simulink model "KalmanFilter_Lateral"  (R2016b)
settings: Solver=VariableStepAuto  StartTime=0.0  StopTime=100  RelTol=1e-3
undefined symbols (not defined in the file or in its folder): A_lat, B_lat, C_lat, Continuous, D_lat, Time
libraries: ctrlSharedLib x1
settings Model: Creator=yashm  LastModifiedBy=yashm

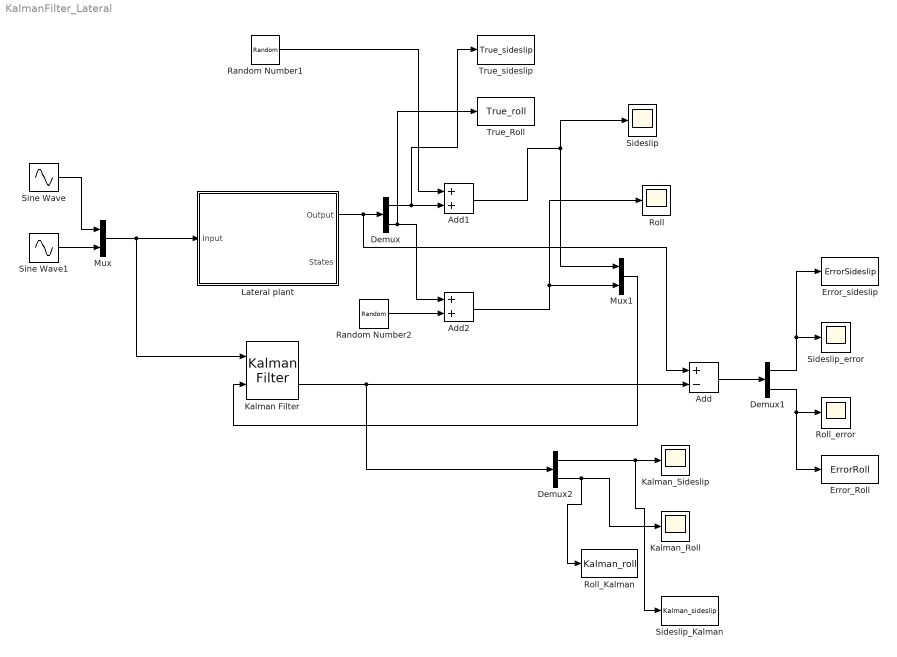
== system KalmanFilter_Lateral ==
  Add : Sum  Inputs=+-
  Add1 : Sum
  Add2 : Sum
  Demux : Demux  Outputs=2
  Demux1 : Demux  Outputs=2
  Demux2 : Demux  Outputs=2
  Error_Roll : ToWorkspace  VariableName=ErrorRoll  SampleTime=0.001
      settings: Save2DSignal=2-D array (concatenate along first dimension)
  Error_sideslip : ToWorkspace  VariableName=ErrorSideslip  SampleTime=0.001
      settings: Save2DSignal=2-D array (concatenate along first dimension)
  Kalman Filter : ctrlSharedLib/Kalman Filter  TimeDomain=Continuous-Time  UseCurrentEstimator=on  ModelSource=Individual A, B, C, D matrices  ModelSourceVariable=ss(0.95,1,1,0,1)  A=A_lat  B=B_lat  C=C_lat  D=D_lat  NumberOfStates=1  NumberOfInputs=1  NumberOfOutputs=1  InitialEstimateSource=Dialog  X0=0  P0=10  UseK=off  UseGH=off  NumberOfProcessNoiseInputs=1  G=1  TimeInvariantG=on  H=0  TimeInvariantH=on  Q=1  TimeInvariantQ=on  R=[1 0;0 1]  TimeInvariantR=on  N=0  TimeInvariantN=on  AddInputPort=on  AddEnablePort=off  ExternalReset=none  OutputEstimatedY=on  OutputP=off  Ts=-1
  Kalman_Roll : Scope
  Kalman_Sideslip : Scope
  "Lateral plant " : Subsystem
  Mux : Mux  Inputs=2
  Mux1 : Mux  Inputs=2
  Random Number1 : RandomNumber  Variance=0.01  SampleTime=0.0001
  Random Number2 : RandomNumber  Variance=3  SampleTime=0.0001
  Roll : Scope
  Roll_Kalman : ToWorkspace  VariableName=Kalman_roll  SampleTime=0.001
      settings: Save2DSignal=2-D array (concatenate along first dimension)
  Roll_error : Scope
  Sideslip : Scope
  Sideslip_Kalman : ToWorkspace  VariableName=Kalman_sideslip  SampleTime=0.001
      settings: Save2DSignal=2-D array (concatenate along first dimension)
  Sideslip_error : Scope
  Sine Wave : Sin  Frequency=15  SampleTime=0
  Sine Wave1 : Sin  Frequency=15  SampleTime=0
  True_Roll : ToWorkspace  VariableName=True_roll  SampleTime=0.001
      settings: Save2DSignal=2-D array (concatenate along first dimension)
  True_sideslip : ToWorkspace  VariableName=True_sideslip  SampleTime=0.001
      settings: Save2DSignal=2-D array (concatenate along first dimension)
  wires:
  "Lateral plant "/1(Output) -> Add/1, Demux/1
  Demux/1 -> True_sideslip/1, Add1/2
  Random Number1/1 -> Add1/1
  Add1/1 -> Mux1/1, Sideslip/1
  Sine Wave1/1 -> Mux/2
  Sine Wave/1 -> Mux/1
  Mux/1 -> Kalman Filter/1, "Lateral plant "/1(Input)
  Kalman Filter/2 -> Demux2/1, Add/2
  Random Number2/1 -> Add2/2
  Demux/2 -> True_Roll/1, Add2/1
  Add2/1 -> Mux1/2, Roll/1
  Mux1/1 -> Kalman Filter/2
  Add/1 -> Demux1/1
  Demux2/1 -> Sideslip_Kalman/1, Kalman_Sideslip/1
  Demux2/2 -> Roll_Kalman/1, Kalman_Roll/1
  Demux1/2 -> Error_Roll/1, Roll_error/1
  Demux1/1 -> Error_sideslip/1, Sideslip_error/1

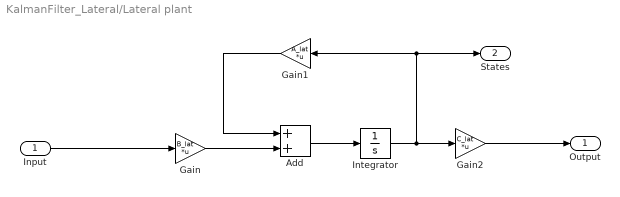
== system KalmanFilter_Lateral/Lateral plant  ==
  Input : Inport
  Add : Sum
  Gain : Gain  Gain=B_lat  Multiplication=Matrix(K*u)
  Gain1 : Gain  Gain=A_lat  Multiplication=Matrix(K*u)
  Gain2 : Gain  Gain=C_lat  Multiplication=Matrix(K*u)
  Integrator : Integrator
  Output : Outport
  States : Outport  Port=2
  wires:
  Input/1 -> Gain/1
  Integrator/1 -> States/1, Gain1/1, Gain2/1
  Gain/1 -> Add/2
  Gain1/1 -> Add/1
  Gain2/1 -> Output/1
  Add/1 -> Integrator/1
